simulink model "Extended_Model_1_1"  (R2024a)
settings: Solver=ode15s  StartTime=0.0  StopTime=100  FixedStep=0.0001  MaxStep=0.01  RelTol=1e-3  AbsTol=1e-3  EnableMultiTasking=on
model workspace (MATLAB code in the model file):
  | F_load_x= 2e3; %[N]
  | F_load_y= 1e4; %[N]
  | 
  | d=0.01;   %[m]
  | l=1;      %[m]
  | L=l;      %[m] Node distance
  | H=L*cos(pi/6); %[m] Node distance
  | 
  | Density=7800; %[kg/m^3]
  | E=210;   %[GPa]
  | G=79;    %[GPa]
  | bm=0.01; %[1/s]  Default
  | bk=0.01; %[s] Default
  | 
  | b_rj=1; %[N*m*s/rad] Damp.Coef.Revolut joints
  | 
  | Size_frame=30; %[pixel]
undefined symbols (not defined in the file): F_x, F_y, X, Y, Z
libraries: sm_lib x317, nesl_utility x64, fl_lib x6, simulink x1
(part 7 of 9)

== system Extended_Model_1_1/Subsystem4/Beam_4 ==
  note: Beam_D
  con : Inport
  Beam : sm_lib/Body Elements/Flexible Bodies/Beams/Flexible Cylindrical Beam  SectionType=Solid  Radius=d/2  RadiusUnits=m  Thickness=1  ThicknessUnits=mm  Length=l  LengthUnits=m  StiffnessAndInertiaType=CalculateFromGeometry  Density=Density  DensityUnits=kg/m^3  ModuliType=YoungsShear  YoungsModulus=E  YoungsModulusUnits=GPa  PoissonsRatio=0.28  ShearModulus=G  ShearModulusUnits=GPa  GeometricCentroid=[0 0]  GeometricCentroidUnits=m  BendingCentroid=[0 0]  BendingCentroidUnits=m  ShearCenter=[0 0]  ShearCenterUnits=m  AxialRigidity=1  AxialRigidityUnits=Pa*m^2  FlexuralRigidity=[1 1]  FlexuralRigidityUnits=Pa*m^4  CrossFlexuralRigidity=0  CrossFlexuralRigidityUnits=Pa*m^4  TorsionalRigidity=1  TorsionalRigidityUnits=Pa*m^4  CenterOfMass=[0 0]  CenterOfMassUnits=m  MassPerUnitLength=1  MassPerUnitLengthUnits=kg/m  MassMomentOfInertiaDensity=[1 1]  MassMomentOfInertiaDensityUnits=kg*m  MassProductOfInertiaDensity=0  MassProductOfInertiaDensityUnits=kg*m  DampingType=Proportional  ProportionalDampingAlpha=bm  ProportionalDampingAlphaUnits=1/s  ProportionalDampingBeta=bk  ProportionalDampingBetaUnits=s  UniformModalDampingRatio=0.01  NumElements=1  ReductionType=None  NumRetainedModes=1  GraphicType=FromGeometry  GraphicVisPropType=SimpleVisualProperties  GraphicDiffuseColor=[0.5 0.5 0.5]  GraphicOpacity=1.0  GraphicSpecularColor=[0.5 0.5 0.5 1.0]  GraphicAmbientColor=[0.15 0.15 0.15 1.0]  GraphicEmissiveColor=[0.0 0.0 0.0 1.0]  GraphicShininess=75  DoExposeZminFrame=on  DoExposeZmaxFrame=on  SerializedFrames=<Frames/>
      settings: AttributesFormatString=%<Description>
  Dot Product : DotProduct  OutDataTypeStr=Inherit: Inherit via internal rule
  Interpreted MATLAB Function : MATLABFcn  Description=u(3)  MATLABFcn=u(3)
      settings: AttributesFormatString=%<Description>
  PS-Simulink Converter6 : nesl_utility/PS-Simulink Converter  PhysicalDomain=network_engine_domain  SubClassName=ps_output  LeftPortType=input  RightPortType=output  PseudoPeriodic=off  Frequencies=[]  VectorFormat=inherit  Unit=1  AffineConversion=off
  Rigid Transform1 : sm_lib/Frames and Transforms/Rigid Transform  RotationMethod=StandardAxis  FollAlignAxisA=+X  BaseAlignAxisA=+Y  FollAlignAxisB=+Y  BaseAlignAxisB=+Z  RotationStandardAxis=+Y  RotationAngle=90  RotationAngleUnits=deg  RotationArbitraryAxis=[0 0 1]  RotationSequenceAxes=FollowerAxes  RotationSequence=XYX  RotationSequenceAngles=[0 0 0]  RotationSequenceAnglesUnits=deg  RotationMatrix=[1 0 0; 0 1 0; 0 0 1]  Quaternion=[1 0 0 0]  TranslationMethod=None  TranslationCartesianOffset=[0 0 0]  TranslationCartesianOffsetUnits=m  TranslationStandardAxis=+Z  TranslationStandardOffset=0  TranslationStandardOffsetUnits=m  TranslationROffset=0  TranslationROffsetUnits=m  TranslationThetaOffset=0  TranslationThetaOffsetUnits=deg  TranslationZOffset=0  TranslationZOffsetUnits=m
      settings: AttributesFormatString=|
      | %<RotationStandardAxis>
      | %<RotationAngle> deg
  Rigid Transform2 : sm_lib/Frames and Transforms/Rigid Transform  RotationMethod=StandardAxis  FollAlignAxisA=+X  BaseAlignAxisA=+Y  FollAlignAxisB=+Y  BaseAlignAxisB=+Z  RotationStandardAxis=+Y  RotationAngle=-90  RotationAngleUnits=deg  RotationArbitraryAxis=[0 0 1]  RotationSequenceAxes=FollowerAxes  RotationSequence=XYX  RotationSequenceAngles=[0 0 0]  RotationSequenceAnglesUnits=deg  RotationMatrix=[1 0 0; 0 1 0; 0 0 1]  Quaternion=[1 0 0 0]  TranslationMethod=None  TranslationCartesianOffset=[0 0 0]  TranslationCartesianOffsetUnits=m  TranslationStandardAxis=+Z  TranslationStandardOffset=0  TranslationStandardOffsetUnits=m  TranslationROffset=0  TranslationROffsetUnits=m  TranslationThetaOffset=0  TranslationThetaOffsetUnits=deg  TranslationZOffset=0  TranslationZOffsetUnits=m
      settings: AttributesFormatString=|
      | %<RotationStandardAxis>
      | %<RotationAngle> deg
  Weld Joint2 : sm_lib/Joints/Weld Joint  Description=|  JointMode=Normal  CompositeWrenchDir=FollowerOnBase  CompositeWrenchFrame=BaseFrame  SenseConstraintForce=off  SenseConstraintTorque=off  SenseTotalForce=on  SenseTotalTorque=off
      | Total force
      | sensing
      settings: AttributesFormatString=%<Description>
  B : PMIOPort  Side=Left
  F : PMIOPort  Port=2  Side=Right
  Ni : Outport
  wires:
  Interpreted MATLAB Function/1 -> Dot Product/1
  Dot Product/1 -> Ni/1
  con/1 -> Dot Product/2
  PS-Simulink Converter6/1 -> Interpreted MATLAB Function/1
  connections:
  Weld Joint2/RConn2 -- PS-Simulink Converter6/LConn1
  Rigid Transform1/LConn1 -- B/RConn1
  Beam/RConn1 -- Rigid Transform2/LConn1
  Rigid Transform2/RConn1 -- F/RConn1
  Weld Joint2/LConn1 -- Rigid Transform1/RConn1
  Beam/LConn1 -- Weld Joint2/RConn1

== system Extended_Model_1_1/Subsystem4/Subsystem ==
  Point Cloud1 : sm_lib/Curves and Surfaces/Point Cloud  Description=|  CoordinatesMatrix=[0 0 0]  CoordinatesMatrixUnits=m  GraphicType=MarkerCloud  GraphicSphereRadius=d/2  GraphicSphereRadiusUnits=m  GraphicVisPropType=SimpleVisualProperties  GraphicDiffuseColor=[0.5 0.5 0.5]  GraphicOpacity=1  GraphicSpecularColor=[0.5 0.5 0.5 1.0]  GraphicAmbientColor=[0.15 0.15 0.15 1.0]  GraphicEmissiveColor=[0.0 0.0 0.0 1.0]  GraphicShininess=75
      | Graphic
      | sphere
      settings: AttributesFormatString=%<Description>
  Point1 : sm_lib/Curves and Surfaces/Point  Description=|  GraphicType=Marker  MarkerShape=Frame  MarkerSize=Size_frame  GraphicVisPropType=SimpleVisualProperties  GraphicDiffuseColor=[0 1 0]  GraphicOpacity=1.0  GraphicSpecularColor=[0.5 0.5 0.5 1.0]  GraphicAmbientColor=[0.15 0.15 0.15 1.0]  GraphicEmissiveColor=[0.0 0.0 0.0 1.0]  GraphicShininess=75
      | Frame
      | visualization
      settings: AttributesFormatString=%<Description>
  Frame : PMIOPort  Side=Left
  connections:
  Point Cloud1/LConn1 -- Frame/RConn1 -- Point1/LConn1

== system Extended_Model_1_1/Subsystem4/Subsystem1 ==
  Point Cloud1 : sm_lib/Curves and Surfaces/Point Cloud  Description=|  CoordinatesMatrix=[0 0 0]  CoordinatesMatrixUnits=m  GraphicType=MarkerCloud  GraphicSphereRadius=d/2  GraphicSphereRadiusUnits=m  GraphicVisPropType=SimpleVisualProperties  GraphicDiffuseColor=[0.5 0.5 0.5]  GraphicOpacity=1  GraphicSpecularColor=[0.5 0.5 0.5 1.0]  GraphicAmbientColor=[0.15 0.15 0.15 1.0]  GraphicEmissiveColor=[0.0 0.0 0.0 1.0]  GraphicShininess=75
      | Graphic
      | sphere
      settings: AttributesFormatString=%<Description>
  Point1 : sm_lib/Curves and Surfaces/Point  Description=|  GraphicType=Marker  MarkerShape=Frame  MarkerSize=Size_frame  GraphicVisPropType=SimpleVisualProperties  GraphicDiffuseColor=[0 1 0]  GraphicOpacity=1.0  GraphicSpecularColor=[0.5 0.5 0.5 1.0]  GraphicAmbientColor=[0.15 0.15 0.15 1.0]  GraphicEmissiveColor=[0.0 0.0 0.0 1.0]  GraphicShininess=75
      | Frame
      | visualization
      settings: AttributesFormatString=%<Description>
  Frame : PMIOPort  Side=Left
  connections:
  Point Cloud1/LConn1 -- Frame/RConn1 -- Point1/LConn1

== system Extended_Model_1_1/Subsystem4/Subsystem2 ==
  Point Cloud1 : sm_lib/Curves and Surfaces/Point Cloud  Description=|  CoordinatesMatrix=[0 0 0]  CoordinatesMatrixUnits=m  GraphicType=MarkerCloud  GraphicSphereRadius=d/2  GraphicSphereRadiusUnits=m  GraphicVisPropType=SimpleVisualProperties  GraphicDiffuseColor=[0.5 0.5 0.5]  GraphicOpacity=1  GraphicSpecularColor=[0.5 0.5 0.5 1.0]  GraphicAmbientColor=[0.15 0.15 0.15 1.0]  GraphicEmissiveColor=[0.0 0.0 0.0 1.0]  GraphicShininess=75
      | Graphic
      | sphere
      settings: AttributesFormatString=%<Description>
  Point1 : sm_lib/Curves and Surfaces/Point  Description=|  GraphicType=Marker  MarkerShape=Frame  MarkerSize=Size_frame  GraphicVisPropType=SimpleVisualProperties  GraphicDiffuseColor=[0 1 0]  GraphicOpacity=1.0  GraphicSpecularColor=[0.5 0.5 0.5 1.0]  GraphicAmbientColor=[0.15 0.15 0.15 1.0]  GraphicEmissiveColor=[0.0 0.0 0.0 1.0]  GraphicShininess=75
      | Frame
      | visualization
      settings: AttributesFormatString=%<Description>
  Frame : PMIOPort  Side=Left
  connections:
  Point1/LConn1 -- Frame/RConn1 -- Point Cloud1/LConn1

== system Extended_Model_1_1/Subsystem5/Beam_1 ==
  note: Beam_A
  con : Inport
  Dot Product : DotProduct  OutDataTypeStr=Inherit: Inherit via internal rule
  Flexible Cylindrical Beam1 : sm_lib/Body Elements/Flexible Bodies/Beams/Flexible Cylindrical Beam  SectionType=Solid  Radius=d/2  RadiusUnits=m  Thickness=1  ThicknessUnits=mm  Length=l  LengthUnits=m  StiffnessAndInertiaType=CalculateFromGeometry  Density=Density  DensityUnits=kg/m^3  ModuliType=YoungsShear  YoungsModulus=E  YoungsModulusUnits=GPa  PoissonsRatio=0.28  ShearModulus=G  ShearModulusUnits=GPa  GeometricCentroid=[0 0]  GeometricCentroidUnits=m  BendingCentroid=[0 0]  BendingCentroidUnits=m  ShearCenter=[0 0]  ShearCenterUnits=m  AxialRigidity=1  AxialRigidityUnits=Pa*m^2  FlexuralRigidity=[1 1]  FlexuralRigidityUnits=Pa*m^4  CrossFlexuralRigidity=0  CrossFlexuralRigidityUnits=Pa*m^4  TorsionalRigidity=1  TorsionalRigidityUnits=Pa*m^4  CenterOfMass=[0 0]  CenterOfMassUnits=m  MassPerUnitLength=1  MassPerUnitLengthUnits=kg/m  MassMomentOfInertiaDensity=[1 1]  MassMomentOfInertiaDensityUnits=kg*m  MassProductOfInertiaDensity=0  MassProductOfInertiaDensityUnits=kg*m  DampingType=Proportional  ProportionalDampingAlpha=bm  ProportionalDampingAlphaUnits=1/s  ProportionalDampingBeta=bk  ProportionalDampingBetaUnits=s  UniformModalDampingRatio=0.01  NumElements=1  ReductionType=None  NumRetainedModes=1  GraphicType=FromGeometry  GraphicVisPropType=SimpleVisualProperties  GraphicDiffuseColor=[0.5 0.5 0.5]  GraphicOpacity=1.0  GraphicSpecularColor=[0.5 0.5 0.5 1.0]  GraphicAmbientColor=[0.15 0.15 0.15 1.0]  GraphicEmissiveColor=[0.0 0.0 0.0 1.0]  GraphicShininess=75  DoExposeZminFrame=on  DoExposeZmaxFrame=on  SerializedFrames=<Frames/>
      settings: AttributesFormatString=%<Description>
  Interpreted MATLAB Function : MATLABFcn  Description=u(3)  MATLABFcn=u(3)
      settings: AttributesFormatString=%<Description>
  PS-Simulink Converter6 : nesl_utility/PS-Simulink Converter  PhysicalDomain=network_engine_domain  SubClassName=ps_output  LeftPortType=input  RightPortType=output  PseudoPeriodic=off  Frequencies=[]  VectorFormat=inherit  Unit=1  AffineConversion=off
  Rigid Transform1 : sm_lib/Frames and Transforms/Rigid Transform  RotationMethod=StandardAxis  FollAlignAxisA=+X  BaseAlignAxisA=+Y  FollAlignAxisB=+Y  BaseAlignAxisB=+Z  RotationStandardAxis=+Y  RotationAngle=90  RotationAngleUnits=deg  RotationArbitraryAxis=[0 0 1]  RotationSequenceAxes=FollowerAxes  RotationSequence=XYX  RotationSequenceAngles=[0 0 0]  RotationSequenceAnglesUnits=deg  RotationMatrix=[1 0 0; 0 1 0; 0 0 1]  Quaternion=[1 0 0 0]  TranslationMethod=None  TranslationCartesianOffset=[0 0 0]  TranslationCartesianOffsetUnits=m  TranslationStandardAxis=+Z  TranslationStandardOffset=0  TranslationStandardOffsetUnits=m  TranslationROffset=0  TranslationROffsetUnits=m  TranslationThetaOffset=0  TranslationThetaOffsetUnits=deg  TranslationZOffset=0  TranslationZOffsetUnits=m
      settings: AttributesFormatString=|
      | %<RotationStandardAxis>
      | %<RotationAngle> deg
  Rigid Transform2 : sm_lib/Frames and Transforms/Rigid Transform  RotationMethod=StandardAxis  FollAlignAxisA=+X  BaseAlignAxisA=+Y  FollAlignAxisB=+Y  BaseAlignAxisB=+Z  RotationStandardAxis=+Y  RotationAngle=-90  RotationAngleUnits=deg  RotationArbitraryAxis=[0 0 1]  RotationSequenceAxes=FollowerAxes  RotationSequence=XYX  RotationSequenceAngles=[0 0 0]  RotationSequenceAnglesUnits=deg  RotationMatrix=[1 0 0; 0 1 0; 0 0 1]  Quaternion=[1 0 0 0]  TranslationMethod=None  TranslationCartesianOffset=[0 0 0]  TranslationCartesianOffsetUnits=m  TranslationStandardAxis=+Z  TranslationStandardOffset=0  TranslationStandardOffsetUnits=m  TranslationROffset=0  TranslationROffsetUnits=m  TranslationThetaOffset=0  TranslationThetaOffsetUnits=deg  TranslationZOffset=0  TranslationZOffsetUnits=m
      settings: AttributesFormatString=|
      | %<RotationStandardAxis>
      | %<RotationAngle> deg
  Weld Joint2 : sm_lib/Joints/Weld Joint  Description=|  JointMode=Normal  CompositeWrenchDir=FollowerOnBase  CompositeWrenchFrame=BaseFrame  SenseConstraintForce=off  SenseConstraintTorque=off  SenseTotalForce=on  SenseTotalTorque=off
      | Total force
      | sensing
      settings: AttributesFormatString=%<Description>
  B : PMIOPort  Side=Left
  F : PMIOPort  Port=2  Side=Right
  Ni : Outport
  wires:
  Interpreted MATLAB Function/1 -> Dot Product/1
  Dot Product/1 -> Ni/1
  PS-Simulink Converter6/1 -> Interpreted MATLAB Function/1
  con/1 -> Dot Product/2
  connections:
  Weld Joint2/LConn1 -- Rigid Transform1/RConn1
  Flexible Cylindrical Beam1/LConn1 -- Weld Joint2/RConn1
  Rigid Transform1/LConn1 -- B/RConn1
  Rigid Transform2/RConn1 -- F/RConn1
  Flexible Cylindrical Beam1/RConn1 -- Rigid Transform2/LConn1
  Weld Joint2/RConn2 -- PS-Simulink Converter6/LConn1

== system Extended_Model_1_1/Subsystem5/Beam_2 ==
  note: Beam_B
  con : Inport
  Dot Product : DotProduct  OutDataTypeStr=Inherit: Inherit via internal rule
  Flexible Cylindrical Beam1 : sm_lib/Body Elements/Flexible Bodies/Beams/Flexible Cylindrical Beam  SectionType=Solid  Radius=d/2  RadiusUnits=m  Thickness=1  ThicknessUnits=mm  Length=l  LengthUnits=m  StiffnessAndInertiaType=CalculateFromGeometry  Density=Density  DensityUnits=kg/m^3  ModuliType=YoungsShear  YoungsModulus=E  YoungsModulusUnits=GPa  PoissonsRatio=0.28  ShearModulus=G  ShearModulusUnits=GPa  GeometricCentroid=[0 0]  GeometricCentroidUnits=m  BendingCentroid=[0 0]  BendingCentroidUnits=m  ShearCenter=[0 0]  ShearCenterUnits=m  AxialRigidity=1  AxialRigidityUnits=Pa*m^2  FlexuralRigidity=[1 1]  FlexuralRigidityUnits=Pa*m^4  CrossFlexuralRigidity=0  CrossFlexuralRigidityUnits=Pa*m^4  TorsionalRigidity=1  TorsionalRigidityUnits=Pa*m^4  CenterOfMass=[0 0]  CenterOfMassUnits=m  MassPerUnitLength=1  MassPerUnitLengthUnits=kg/m  MassMomentOfInertiaDensity=[1 1]  MassMomentOfInertiaDensityUnits=kg*m  MassProductOfInertiaDensity=0  MassProductOfInertiaDensityUnits=kg*m  DampingType=Proportional  ProportionalDampingAlpha=bm  ProportionalDampingAlphaUnits=1/s  ProportionalDampingBeta=bk  ProportionalDampingBetaUnits=s  UniformModalDampingRatio=0.01  NumElements=1  ReductionType=None  NumRetainedModes=1  GraphicType=FromGeometry  GraphicVisPropType=SimpleVisualProperties  GraphicDiffuseColor=[0.5 0.5 0.5]  GraphicOpacity=1.0  GraphicSpecularColor=[0.5 0.5 0.5 1.0]  GraphicAmbientColor=[0.15 0.15 0.15 1.0]  GraphicEmissiveColor=[0.0 0.0 0.0 1.0]  GraphicShininess=75  DoExposeZminFrame=on  DoExposeZmaxFrame=on  SerializedFrames=<Frames/>
      settings: AttributesFormatString=%<Description>
  Interpreted MATLAB Function : MATLABFcn  Description=u(3)  MATLABFcn=u(3)
      settings: AttributesFormatString=%<Description>
  PS-Simulink Converter6 : nesl_utility/PS-Simulink Converter  PhysicalDomain=network_engine_domain  SubClassName=ps_output  LeftPortType=input  RightPortType=output  PseudoPeriodic=off  Frequencies=[]  VectorFormat=inherit  Unit=1  AffineConversion=off
  Rigid Transform1 : sm_lib/Frames and Transforms/Rigid Transform  RotationMethod=StandardAxis  FollAlignAxisA=+X  BaseAlignAxisA=+Y  FollAlignAxisB=+Y  BaseAlignAxisB=+Z  RotationStandardAxis=+Y  RotationAngle=90  RotationAngleUnits=deg  RotationArbitraryAxis=[0 0 1]  RotationSequenceAxes=FollowerAxes  RotationSequence=XYX  RotationSequenceAngles=[0 0 0]  RotationSequenceAnglesUnits=deg  RotationMatrix=[1 0 0; 0 1 0; 0 0 1]  Quaternion=[1 0 0 0]  TranslationMethod=None  TranslationCartesianOffset=[0 0 0]  TranslationCartesianOffsetUnits=m  TranslationStandardAxis=+Z  TranslationStandardOffset=0  TranslationStandardOffsetUnits=m  TranslationROffset=0  TranslationROffsetUnits=m  TranslationThetaOffset=0  TranslationThetaOffsetUnits=deg  TranslationZOffset=0  TranslationZOffsetUnits=m
      settings: AttributesFormatString=|
      | %<RotationStandardAxis>
      | %<RotationAngle> deg
  Rigid Transform2 : sm_lib/Frames and Transforms/Rigid Transform  RotationMethod=StandardAxis  FollAlignAxisA=+X  BaseAlignAxisA=+Y  FollAlignAxisB=+Y  BaseAlignAxisB=+Z  RotationStandardAxis=+Y  RotationAngle=-90  RotationAngleUnits=deg  RotationArbitraryAxis=[0 0 1]  RotationSequenceAxes=FollowerAxes  RotationSequence=XYX  RotationSequenceAngles=[0 0 0]  RotationSequenceAnglesUnits=deg  RotationMatrix=[1 0 0; 0 1 0; 0 0 1]  Quaternion=[1 0 0 0]  TranslationMethod=None  TranslationCartesianOffset=[0 0 0]  TranslationCartesianOffsetUnits=m  TranslationStandardAxis=+Z  TranslationStandardOffset=0  TranslationStandardOffsetUnits=m  TranslationROffset=0  TranslationROffsetUnits=m  TranslationThetaOffset=0  TranslationThetaOffsetUnits=deg  TranslationZOffset=0  TranslationZOffsetUnits=m
      settings: AttributesFormatString=|
      | %<RotationStandardAxis>
      | %<RotationAngle> deg
  Weld Joint2 : sm_lib/Joints/Weld Joint  Description=|  JointMode=Normal  CompositeWrenchDir=FollowerOnBase  CompositeWrenchFrame=BaseFrame  SenseConstraintForce=off  SenseConstraintTorque=off  SenseTotalForce=on  SenseTotalTorque=off
      | Total force
      | sensing
      settings: AttributesFormatString=%<Description>
  B : PMIOPort  Side=Left
  F : PMIOPort  Port=2  Side=Right
  Ni : Outport
  wires:
  con/1 -> Dot Product/2
  PS-Simulink Converter6/1 -> Interpreted MATLAB Function/1
  Dot Product/1 -> Ni/1
  Interpreted MATLAB Function/1 -> Dot Product/1
  connections:
  Weld Joint2/RConn2 -- PS-Simulink Converter6/LConn1
  Flexible Cylindrical Beam1/RConn1 -- Rigid Transform2/LConn1
  Rigid Transform2/RConn1 -- F/RConn1
  Rigid Transform1/LConn1 -- B/RConn1
  Flexible Cylindrical Beam1/LConn1 -- Weld Joint2/RConn1
  Weld Joint2/LConn1 -- Rigid Transform1/RConn1

== system Extended_Model_1_1/Subsystem5/Beam_3 ==
  note: Beam_C
  con : Inport
  Beam : sm_lib/Body Elements/Flexible Bodies/Beams/Flexible Cylindrical Beam  SectionType=Solid  Radius=d/2  RadiusUnits=m  Thickness=1  ThicknessUnits=mm  Length=l  LengthUnits=m  StiffnessAndInertiaType=CalculateFromGeometry  Density=Density  DensityUnits=kg/m^3  ModuliType=YoungsShear  YoungsModulus=E  YoungsModulusUnits=GPa  PoissonsRatio=0.28  ShearModulus=G  ShearModulusUnits=GPa  GeometricCentroid=[0 0]  GeometricCentroidUnits=m  BendingCentroid=[0 0]  BendingCentroidUnits=m  ShearCenter=[0 0]  ShearCenterUnits=m  AxialRigidity=1  AxialRigidityUnits=Pa*m^2  FlexuralRigidity=[1 1]  FlexuralRigidityUnits=Pa*m^4  CrossFlexuralRigidity=0  CrossFlexuralRigidityUnits=Pa*m^4  TorsionalRigidity=1  TorsionalRigidityUnits=Pa*m^4  CenterOfMass=[0 0]  CenterOfMassUnits=m  MassPerUnitLength=1  MassPerUnitLengthUnits=kg/m  MassMomentOfInertiaDensity=[1 1]  MassMomentOfInertiaDensityUnits=kg*m  MassProductOfInertiaDensity=0  MassProductOfInertiaDensityUnits=kg*m  DampingType=Proportional  ProportionalDampingAlpha=bm  ProportionalDampingAlphaUnits=1/s  ProportionalDampingBeta=bk  ProportionalDampingBetaUnits=s  UniformModalDampingRatio=0.01  NumElements=1  ReductionType=None  NumRetainedModes=1  GraphicType=FromGeometry  GraphicVisPropType=SimpleVisualProperties  GraphicDiffuseColor=[0.5 0.5 0.5]  GraphicOpacity=1.0  GraphicSpecularColor=[0.5 0.5 0.5 1.0]  GraphicAmbientColor=[0.15 0.15 0.15 1.0]  GraphicEmissiveColor=[0.0 0.0 0.0 1.0]  GraphicShininess=75  DoExposeZminFrame=on  DoExposeZmaxFrame=on  SerializedFrames=<Frames/>
      settings: AttributesFormatString=%<Description>
  Dot Product : DotProduct  OutDataTypeStr=Inherit: Inherit via internal rule
  Interpreted MATLAB Function : MATLABFcn  Description=u(3)  MATLABFcn=u(3)
      settings: AttributesFormatString=%<Description>
  PS-Simulink Converter6 : nesl_utility/PS-Simulink Converter  PhysicalDomain=network_engine_domain  SubClassName=ps_output  LeftPortType=input  RightPortType=output  PseudoPeriodic=off  Frequencies=[]  VectorFormat=inherit  Unit=1  AffineConversion=off
  Rigid Transform1 : sm_lib/Frames and Transforms/Rigid Transform  RotationMethod=StandardAxis  FollAlignAxisA=+X  BaseAlignAxisA=+Y  FollAlignAxisB=+Y  BaseAlignAxisB=+Z  RotationStandardAxis=+Y  RotationAngle=90  RotationAngleUnits=deg  RotationArbitraryAxis=[0 0 1]  RotationSequenceAxes=FollowerAxes  RotationSequence=XYX  RotationSequenceAngles=[0 0 0]  RotationSequenceAnglesUnits=deg  RotationMatrix=[1 0 0; 0 1 0; 0 0 1]  Quaternion=[1 0 0 0]  TranslationMethod=None  TranslationCartesianOffset=[0 0 0]  TranslationCartesianOffsetUnits=m  TranslationStandardAxis=+Z  TranslationStandardOffset=0  TranslationStandardOffsetUnits=m  TranslationROffset=0  TranslationROffsetUnits=m  TranslationThetaOffset=0  TranslationThetaOffsetUnits=deg  TranslationZOffset=0  TranslationZOffsetUnits=m
      settings: AttributesFormatString=|
      | %<RotationStandardAxis>
      | %<RotationAngle> deg
  Rigid Transform2 : sm_lib/Frames and Transforms/Rigid Transform  RotationMethod=StandardAxis  FollAlignAxisA=+X  BaseAlignAxisA=+Y  FollAlignAxisB=+Y  BaseAlignAxisB=+Z  RotationStandardAxis=+Y  RotationAngle=-90  RotationAngleUnits=deg  RotationArbitraryAxis=[0 0 1]  RotationSequenceAxes=FollowerAxes  RotationSequence=XYX  RotationSequenceAngles=[0 0 0]  RotationSequenceAnglesUnits=deg  RotationMatrix=[1 0 0; 0 1 0; 0 0 1]  Quaternion=[1 0 0 0]  TranslationMethod=None  TranslationCartesianOffset=[0 0 0]  TranslationCartesianOffsetUnits=m  TranslationStandardAxis=+Z  TranslationStandardOffset=0  TranslationStandardOffsetUnits=m  TranslationROffset=0  TranslationROffsetUnits=m  TranslationThetaOffset=0  TranslationThetaOffsetUnits=deg  TranslationZOffset=0  TranslationZOffsetUnits=m
      settings: AttributesFormatString=|
      | %<RotationStandardAxis>
      | %<RotationAngle> deg
  Weld Joint2 : sm_lib/Joints/Weld Joint  Description=|  JointMode=Normal  CompositeWrenchDir=FollowerOnBase  CompositeWrenchFrame=BaseFrame  SenseConstraintForce=off  SenseConstraintTorque=off  SenseTotalForce=on  SenseTotalTorque=off
      | Total force
      | sensing
      settings: AttributesFormatString=%<Description>
  B : PMIOPort  Side=Left
  F : PMIOPort  Port=2  Side=Right
  Ni : Outport
  wires:
  PS-Simulink Converter6/1 -> Interpreted MATLAB Function/1
  con/1 -> Dot Product/2
  Dot Product/1 -> Ni/1
  Interpreted MATLAB Function/1 -> Dot Product/1
  connections:
  Beam/LConn1 -- Weld Joint2/RConn1
  Weld Joint2/LConn1 -- Rigid Transform1/RConn1
  Rigid Transform2/RConn1 -- F/RConn1
  Beam/RConn1 -- Rigid Transform2/LConn1
  Rigid Transform1/LConn1 -- B/RConn1
  Weld Joint2/RConn2 -- PS-Simulink Converter6/LConn1

== system Extended_Model_1_1/Subsystem5/Beam_4 ==
  note: Beam_D
  con : Inport
  Beam : sm_lib/Body Elements/Flexible Bodies/Beams/Flexible Cylindrical Beam  SectionType=Solid  Radius=d/2  RadiusUnits=m  Thickness=1  ThicknessUnits=mm  Length=l  LengthUnits=m  StiffnessAndInertiaType=CalculateFromGeometry  Density=Density  DensityUnits=kg/m^3  ModuliType=YoungsShear  YoungsModulus=E  YoungsModulusUnits=GPa  PoissonsRatio=0.28  ShearModulus=G  ShearModulusUnits=GPa  GeometricCentroid=[0 0]  GeometricCentroidUnits=m  BendingCentroid=[0 0]  BendingCentroidUnits=m  ShearCenter=[0 0]  ShearCenterUnits=m  AxialRigidity=1  AxialRigidityUnits=Pa*m^2  FlexuralRigidity=[1 1]  FlexuralRigidityUnits=Pa*m^4  CrossFlexuralRigidity=0  CrossFlexuralRigidityUnits=Pa*m^4  TorsionalRigidity=1  TorsionalRigidityUnits=Pa*m^4  CenterOfMass=[0 0]  CenterOfMassUnits=m  MassPerUnitLength=1  MassPerUnitLengthUnits=kg/m  MassMomentOfInertiaDensity=[1 1]  MassMomentOfInertiaDensityUnits=kg*m  MassProductOfInertiaDensity=0  MassProductOfInertiaDensityUnits=kg*m  DampingType=Proportional  ProportionalDampingAlpha=bm  ProportionalDampingAlphaUnits=1/s  ProportionalDampingBeta=bk  ProportionalDampingBetaUnits=s  UniformModalDampingRatio=0.01  NumElements=1  ReductionType=None  NumRetainedModes=1  GraphicType=FromGeometry  GraphicVisPropType=SimpleVisualProperties  GraphicDiffuseColor=[0.5 0.5 0.5]  GraphicOpacity=1.0  GraphicSpecularColor=[0.5 0.5 0.5 1.0]  GraphicAmbientColor=[0.15 0.15 0.15 1.0]  GraphicEmissiveColor=[0.0 0.0 0.0 1.0]  GraphicShininess=75  DoExposeZminFrame=on  DoExposeZmaxFrame=on  SerializedFrames=<Frames/>
      settings: AttributesFormatString=%<Description>
  Dot Product : DotProduct  OutDataTypeStr=Inherit: Inherit via internal rule
  Interpreted MATLAB Function : MATLABFcn  Description=u(3)  MATLABFcn=u(3)
      settings: AttributesFormatString=%<Description>
  PS-Simulink Converter6 : nesl_utility/PS-Simulink Converter  PhysicalDomain=network_engine_domain  SubClassName=ps_output  LeftPortType=input  RightPortType=output  PseudoPeriodic=off  Frequencies=[]  VectorFormat=inherit  Unit=1  AffineConversion=off
  Rigid Transform1 : sm_lib/Frames and Transforms/Rigid Transform  RotationMethod=StandardAxis  FollAlignAxisA=+X  BaseAlignAxisA=+Y  FollAlignAxisB=+Y  BaseAlignAxisB=+Z  RotationStandardAxis=+Y  RotationAngle=90  RotationAngleUnits=deg  RotationArbitraryAxis=[0 0 1]  RotationSequenceAxes=FollowerAxes  RotationSequence=XYX  RotationSequenceAngles=[0 0 0]  RotationSequenceAnglesUnits=deg  RotationMatrix=[1 0 0; 0 1 0; 0 0 1]  Quaternion=[1 0 0 0]  TranslationMethod=None  TranslationCartesianOffset=[0 0 0]  TranslationCartesianOffsetUnits=m  TranslationStandardAxis=+Z  TranslationStandardOffset=0  TranslationStandardOffsetUnits=m  TranslationROffset=0  TranslationROffsetUnits=m  TranslationThetaOffset=0  TranslationThetaOffsetUnits=deg  TranslationZOffset=0  TranslationZOffsetUnits=m
      settings: AttributesFormatString=|
      | %<RotationStandardAxis>
      | %<RotationAngle> deg
  Rigid Transform2 : sm_lib/Frames and Transforms/Rigid Transform  RotationMethod=StandardAxis  FollAlignAxisA=+X  BaseAlignAxisA=+Y  FollAlignAxisB=+Y  BaseAlignAxisB=+Z  RotationStandardAxis=+Y  RotationAngle=-90  RotationAngleUnits=deg  RotationArbitraryAxis=[0 0 1]  RotationSequenceAxes=FollowerAxes  RotationSequence=XYX  RotationSequenceAngles=[0 0 0]  RotationSequenceAnglesUnits=deg  RotationMatrix=[1 0 0; 0 1 0; 0 0 1]  Quaternion=[1 0 0 0]  TranslationMethod=None  TranslationCartesianOffset=[0 0 0]  TranslationCartesianOffsetUnits=m  TranslationStandardAxis=+Z  TranslationStandardOffset=0  TranslationStandardOffsetUnits=m  TranslationROffset=0  TranslationROffsetUnits=m  TranslationThetaOffset=0  TranslationThetaOffsetUnits=deg  TranslationZOffset=0  TranslationZOffsetUnits=m
      settings: AttributesFormatString=|
      | %<RotationStandardAxis>
      | %<RotationAngle> deg
  Weld Joint2 : sm_lib/Joints/Weld Joint  Description=|  JointMode=Normal  CompositeWrenchDir=FollowerOnBase  CompositeWrenchFrame=BaseFrame  SenseConstraintForce=off  SenseConstraintTorque=off  SenseTotalForce=on  SenseTotalTorque=off
      | Total force
      | sensing
      settings: AttributesFormatString=%<Description>
  B : PMIOPort  Side=Left
  F : PMIOPort  Port=2  Side=Right
  Ni : Outport
  wires:
  PS-Simulink Converter6/1 -> Interpreted MATLAB Function/1
  con/1 -> Dot Product/2
  Dot Product/1 -> Ni/1
  Interpreted MATLAB Function/1 -> Dot Product/1
  connections:
  Beam/LConn1 -- Weld Joint2/RConn1
  Weld Joint2/LConn1 -- Rigid Transform1/RConn1
  Rigid Transform2/RConn1 -- F/RConn1
  Beam/RConn1 -- Rigid Transform2/LConn1
  Rigid Transform1/LConn1 -- B/RConn1
  Weld Joint2/RConn2 -- PS-Simulink Converter6/LConn1

== system Extended_Model_1_1/Subsystem5/Subsystem ==
  Point Cloud1 : sm_lib/Curves and Surfaces/Point Cloud  Description=|  CoordinatesMatrix=[0 0 0]  CoordinatesMatrixUnits=m  GraphicType=MarkerCloud  GraphicSphereRadius=d/2  GraphicSphereRadiusUnits=m  GraphicVisPropType=SimpleVisualProperties  GraphicDiffuseColor=[0.5 0.5 0.5]  GraphicOpacity=1  GraphicSpecularColor=[0.5 0.5 0.5 1.0]  GraphicAmbientColor=[0.15 0.15 0.15 1.0]  GraphicEmissiveColor=[0.0 0.0 0.0 1.0]  GraphicShininess=75
      | Graphic
      | sphere
      settings: AttributesFormatString=%<Description>
  Point1 : sm_lib/Curves and Surfaces/Point  Description=|  GraphicType=Marker  MarkerShape=Frame  MarkerSize=Size_frame  GraphicVisPropType=SimpleVisualProperties  GraphicDiffuseColor=[0 1 0]  GraphicOpacity=1.0  GraphicSpecularColor=[0.5 0.5 0.5 1.0]  GraphicAmbientColor=[0.15 0.15 0.15 1.0]  GraphicEmissiveColor=[0.0 0.0 0.0 1.0]  GraphicShininess=75
      | Frame
      | visualization
      settings: AttributesFormatString=%<Description>
  Frame : PMIOPort  Side=Left
  connections:
  Point1/LConn1 -- Frame/RConn1 -- Point Cloud1/LConn1

== system Extended_Model_1_1/Subsystem5/Subsystem1 ==
  Point Cloud1 : sm_lib/Curves and Surfaces/Point Cloud  Description=|  CoordinatesMatrix=[0 0 0]  CoordinatesMatrixUnits=m  GraphicType=MarkerCloud  GraphicSphereRadius=d/2  GraphicSphereRadiusUnits=m  GraphicVisPropType=SimpleVisualProperties  GraphicDiffuseColor=[0.5 0.5 0.5]  GraphicOpacity=1  GraphicSpecularColor=[0.5 0.5 0.5 1.0]  GraphicAmbientColor=[0.15 0.15 0.15 1.0]  GraphicEmissiveColor=[0.0 0.0 0.0 1.0]  GraphicShininess=75
      | Graphic
      | sphere
      settings: AttributesFormatString=%<Description>
  Point1 : sm_lib/Curves and Surfaces/Point  Description=|  GraphicType=Marker  MarkerShape=Frame  MarkerSize=Size_frame  GraphicVisPropType=SimpleVisualProperties  GraphicDiffuseColor=[0 1 0]  GraphicOpacity=1.0  GraphicSpecularColor=[0.5 0.5 0.5 1.0]  GraphicAmbientColor=[0.15 0.15 0.15 1.0]  GraphicEmissiveColor=[0.0 0.0 0.0 1.0]  GraphicShininess=75
      | Frame
      | visualization
      settings: AttributesFormatString=%<Description>
  Frame : PMIOPort  Side=Left
  connections:
  Point1/LConn1 -- Frame/RConn1 -- Point Cloud1/LConn1

== system Extended_Model_1_1/Subsystem5/Subsystem2 ==
  Point Cloud1 : sm_lib/Curves and Surfaces/Point Cloud  Description=|  CoordinatesMatrix=[0 0 0]  CoordinatesMatrixUnits=m  GraphicType=MarkerCloud  GraphicSphereRadius=d/2  GraphicSphereRadiusUnits=m  GraphicVisPropType=SimpleVisualProperties  GraphicDiffuseColor=[0.5 0.5 0.5]  GraphicOpacity=1  GraphicSpecularColor=[0.5 0.5 0.5 1.0]  GraphicAmbientColor=[0.15 0.15 0.15 1.0]  GraphicEmissiveColor=[0.0 0.0 0.0 1.0]  GraphicShininess=75
      | Graphic
      | sphere
      settings: AttributesFormatString=%<Description>
  Point1 : sm_lib/Curves and Surfaces/Point  Description=|  GraphicType=Marker  MarkerShape=Frame  MarkerSize=Size_frame  GraphicVisPropType=SimpleVisualProperties  GraphicDiffuseColor=[0 1 0]  GraphicOpacity=1.0  GraphicSpecularColor=[0.5 0.5 0.5 1.0]  GraphicAmbientColor=[0.15 0.15 0.15 1.0]  GraphicEmissiveColor=[0.0 0.0 0.0 1.0]  GraphicShininess=75
      | Frame
      | visualization
      settings: AttributesFormatString=%<Description>
  Frame : PMIOPort  Side=Left
  connections:
  Point Cloud1/LConn1 -- Frame/RConn1 -- Point1/LConn1

== system Extended_Model_1_1/Subsystem6/Beam_1 ==
  note: Beam_A
  con : Inport
  Dot Product : DotProduct  OutDataTypeStr=Inherit: Inherit via internal rule
  Flexible Cylindrical Beam1 : sm_lib/Body Elements/Flexible Bodies/Beams/Flexible Cylindrical Beam  SectionType=Solid  Radius=d/2  RadiusUnits=m  Thickness=1  ThicknessUnits=mm  Length=l  LengthUnits=m  StiffnessAndInertiaType=CalculateFromGeometry  Density=Density  DensityUnits=kg/m^3  ModuliType=YoungsShear  YoungsModulus=E  YoungsModulusUnits=GPa  PoissonsRatio=0.28  ShearModulus=G  ShearModulusUnits=GPa  GeometricCentroid=[0 0]  GeometricCentroidUnits=m  BendingCentroid=[0 0]  BendingCentroidUnits=m  ShearCenter=[0 0]  ShearCenterUnits=m  AxialRigidity=1  AxialRigidityUnits=Pa*m^2  FlexuralRigidity=[1 1]  FlexuralRigidityUnits=Pa*m^4  CrossFlexuralRigidity=0  CrossFlexuralRigidityUnits=Pa*m^4  TorsionalRigidity=1  TorsionalRigidityUnits=Pa*m^4  CenterOfMass=[0 0]  CenterOfMassUnits=m  MassPerUnitLength=1  MassPerUnitLengthUnits=kg/m  MassMomentOfInertiaDensity=[1 1]  MassMomentOfInertiaDensityUnits=kg*m  MassProductOfInertiaDensity=0  MassProductOfInertiaDensityUnits=kg*m  DampingType=Proportional  ProportionalDampingAlpha=bm  ProportionalDampingAlphaUnits=1/s  ProportionalDampingBeta=bk  ProportionalDampingBetaUnits=s  UniformModalDampingRatio=0.01  NumElements=1  ReductionType=None  NumRetainedModes=1  GraphicType=FromGeometry  GraphicVisPropType=SimpleVisualProperties  GraphicDiffuseColor=[0.5 0.5 0.5]  GraphicOpacity=1.0  GraphicSpecularColor=[0.5 0.5 0.5 1.0]  GraphicAmbientColor=[0.15 0.15 0.15 1.0]  GraphicEmissiveColor=[0.0 0.0 0.0 1.0]  GraphicShininess=75  DoExposeZminFrame=on  DoExposeZmaxFrame=on  SerializedFrames=<Frames/>
      settings: AttributesFormatString=%<Description>
  Interpreted MATLAB Function : MATLABFcn  Description=u(3)  MATLABFcn=u(3)
      settings: AttributesFormatString=%<Description>
  PS-Simulink Converter6 : nesl_utility/PS-Simulink Converter  PhysicalDomain=network_engine_domain  SubClassName=ps_output  LeftPortType=input  RightPortType=output  PseudoPeriodic=off  Frequencies=[]  VectorFormat=inherit  Unit=1  AffineConversion=off
  Rigid Transform1 : sm_lib/Frames and Transforms/Rigid Transform  RotationMethod=StandardAxis  FollAlignAxisA=+X  BaseAlignAxisA=+Y  FollAlignAxisB=+Y  BaseAlignAxisB=+Z  RotationStandardAxis=+Y  RotationAngle=90  RotationAngleUnits=deg  RotationArbitraryAxis=[0 0 1]  RotationSequenceAxes=FollowerAxes  RotationSequence=XYX  RotationSequenceAngles=[0 0 0]  RotationSequenceAnglesUnits=deg  RotationMatrix=[1 0 0; 0 1 0; 0 0 1]  Quaternion=[1 0 0 0]  TranslationMethod=None  TranslationCartesianOffset=[0 0 0]  TranslationCartesianOffsetUnits=m  TranslationStandardAxis=+Z  TranslationStandardOffset=0  TranslationStandardOffsetUnits=m  TranslationROffset=0  TranslationROffsetUnits=m  TranslationThetaOffset=0  TranslationThetaOffsetUnits=deg  TranslationZOffset=0  TranslationZOffsetUnits=m
      settings: AttributesFormatString=|
      | %<RotationStandardAxis>
      | %<RotationAngle> deg
  Rigid Transform2 : sm_lib/Frames and Transforms/Rigid Transform  RotationMethod=StandardAxis  FollAlignAxisA=+X  BaseAlignAxisA=+Y  FollAlignAxisB=+Y  BaseAlignAxisB=+Z  RotationStandardAxis=+Y  RotationAngle=-90  RotationAngleUnits=deg  RotationArbitraryAxis=[0 0 1]  RotationSequenceAxes=FollowerAxes  RotationSequence=XYX  RotationSequenceAngles=[0 0 0]  RotationSequenceAnglesUnits=deg  RotationMatrix=[1 0 0; 0 1 0; 0 0 1]  Quaternion=[1 0 0 0]  TranslationMethod=None  TranslationCartesianOffset=[0 0 0]  TranslationCartesianOffsetUnits=m  TranslationStandardAxis=+Z  TranslationStandardOffset=0  TranslationStandardOffsetUnits=m  TranslationROffset=0  TranslationROffsetUnits=m  TranslationThetaOffset=0  TranslationThetaOffsetUnits=deg  TranslationZOffset=0  TranslationZOffsetUnits=m
      settings: AttributesFormatString=|
      | %<RotationStandardAxis>
      | %<RotationAngle> deg
  Weld Joint2 : sm_lib/Joints/Weld Joint  Description=|  JointMode=Normal  CompositeWrenchDir=FollowerOnBase  CompositeWrenchFrame=BaseFrame  SenseConstraintForce=off  SenseConstraintTorque=off  SenseTotalForce=on  SenseTotalTorque=off
      | Total force
      | sensing
      settings: AttributesFormatString=%<Description>
  B : PMIOPort  Side=Left
  F : PMIOPort  Port=2  Side=Right
  Ni : Outport
  wires:
  con/1 -> Dot Product/2
  PS-Simulink Converter6/1 -> Interpreted MATLAB Function/1
  Dot Product/1 -> Ni/1
  Interpreted MATLAB Function/1 -> Dot Product/1
  connections:
  Weld Joint2/RConn2 -- PS-Simulink Converter6/LConn1
  Flexible Cylindrical Beam1/RConn1 -- Rigid Transform2/LConn1
  Rigid Transform2/RConn1 -- F/RConn1
  Rigid Transform1/LConn1 -- B/RConn1
  Flexible Cylindrical Beam1/LConn1 -- Weld Joint2/RConn1
  Weld Joint2/LConn1 -- Rigid Transform1/RConn1

== system Extended_Model_1_1/Subsystem6/Beam_2 ==
  note: Beam_B
  con : Inport
  Dot Product : DotProduct  OutDataTypeStr=Inherit: Inherit via internal rule
  Flexible Cylindrical Beam1 : sm_lib/Body Elements/Flexible Bodies/Beams/Flexible Cylindrical Beam  SectionType=Solid  Radius=d/2  RadiusUnits=m  Thickness=1  ThicknessUnits=mm  Length=l  LengthUnits=m  StiffnessAndInertiaType=CalculateFromGeometry  Density=Density  DensityUnits=kg/m^3  ModuliType=YoungsShear  YoungsModulus=E  YoungsModulusUnits=GPa  PoissonsRatio=0.28  ShearModulus=G  ShearModulusUnits=GPa  GeometricCentroid=[0 0]  GeometricCentroidUnits=m  BendingCentroid=[0 0]  BendingCentroidUnits=m  ShearCenter=[0 0]  ShearCenterUnits=m  AxialRigidity=1  AxialRigidityUnits=Pa*m^2  FlexuralRigidity=[1 1]  FlexuralRigidityUnits=Pa*m^4  CrossFlexuralRigidity=0  CrossFlexuralRigidityUnits=Pa*m^4  TorsionalRigidity=1  TorsionalRigidityUnits=Pa*m^4  CenterOfMass=[0 0]  CenterOfMassUnits=m  MassPerUnitLength=1  MassPerUnitLengthUnits=kg/m  MassMomentOfInertiaDensity=[1 1]  MassMomentOfInertiaDensityUnits=kg*m  MassProductOfInertiaDensity=0  MassProductOfInertiaDensityUnits=kg*m  DampingType=Proportional  ProportionalDampingAlpha=bm  ProportionalDampingAlphaUnits=1/s  ProportionalDampingBeta=bk  ProportionalDampingBetaUnits=s  UniformModalDampingRatio=0.01  NumElements=1  ReductionType=None  NumRetainedModes=1  GraphicType=FromGeometry  GraphicVisPropType=SimpleVisualProperties  GraphicDiffuseColor=[0.5 0.5 0.5]  GraphicOpacity=1.0  GraphicSpecularColor=[0.5 0.5 0.5 1.0]  GraphicAmbientColor=[0.15 0.15 0.15 1.0]  GraphicEmissiveColor=[0.0 0.0 0.0 1.0]  GraphicShininess=75  DoExposeZminFrame=on  DoExposeZmaxFrame=on  SerializedFrames=<Frames/>
      settings: AttributesFormatString=%<Description>
  Interpreted MATLAB Function : MATLABFcn  Description=u(3)  MATLABFcn=u(3)
      settings: AttributesFormatString=%<Description>
  PS-Simulink Converter6 : nesl_utility/PS-Simulink Converter  PhysicalDomain=network_engine_domain  SubClassName=ps_output  LeftPortType=input  RightPortType=output  PseudoPeriodic=off  Frequencies=[]  VectorFormat=inherit  Unit=1  AffineConversion=off
  Rigid Transform1 : sm_lib/Frames and Transforms/Rigid Transform  RotationMethod=StandardAxis  FollAlignAxisA=+X  BaseAlignAxisA=+Y  FollAlignAxisB=+Y  BaseAlignAxisB=+Z  RotationStandardAxis=+Y  RotationAngle=90  RotationAngleUnits=deg  RotationArbitraryAxis=[0 0 1]  RotationSequenceAxes=FollowerAxes  RotationSequence=XYX  RotationSequenceAngles=[0 0 0]  RotationSequenceAnglesUnits=deg  RotationMatrix=[1 0 0; 0 1 0; 0 0 1]  Quaternion=[1 0 0 0]  TranslationMethod=None  TranslationCartesianOffset=[0 0 0]  TranslationCartesianOffsetUnits=m  TranslationStandardAxis=+Z  TranslationStandardOffset=0  TranslationStandardOffsetUnits=m  TranslationROffset=0  TranslationROffsetUnits=m  TranslationThetaOffset=0  TranslationThetaOffsetUnits=deg  TranslationZOffset=0  TranslationZOffsetUnits=m
      settings: AttributesFormatString=|
      | %<RotationStandardAxis>
      | %<RotationAngle> deg
  Rigid Transform2 : sm_lib/Frames and Transforms/Rigid Transform  RotationMethod=StandardAxis  FollAlignAxisA=+X  BaseAlignAxisA=+Y  FollAlignAxisB=+Y  BaseAlignAxisB=+Z  RotationStandardAxis=+Y  RotationAngle=-90  RotationAngleUnits=deg  RotationArbitraryAxis=[0 0 1]  RotationSequenceAxes=FollowerAxes  RotationSequence=XYX  RotationSequenceAngles=[0 0 0]  RotationSequenceAnglesUnits=deg  RotationMatrix=[1 0 0; 0 1 0; 0 0 1]  Quaternion=[1 0 0 0]  TranslationMethod=None  TranslationCartesianOffset=[0 0 0]  TranslationCartesianOffsetUnits=m  TranslationStandardAxis=+Z  TranslationStandardOffset=0  TranslationStandardOffsetUnits=m  TranslationROffset=0  TranslationROffsetUnits=m  TranslationThetaOffset=0  TranslationThetaOffsetUnits=deg  TranslationZOffset=0  TranslationZOffsetUnits=m
      settings: AttributesFormatString=|
      | %<RotationStandardAxis>
      | %<RotationAngle> deg
  Weld Joint2 : sm_lib/Joints/Weld Joint  Description=|  JointMode=Normal  CompositeWrenchDir=FollowerOnBase  CompositeWrenchFrame=BaseFrame  SenseConstraintForce=off  SenseConstraintTorque=off  SenseTotalForce=on  SenseTotalTorque=off
      | Total force
      | sensing
      settings: AttributesFormatString=%<Description>
  B : PMIOPort  Side=Left
  F : PMIOPort  Port=2  Side=Right
  Ni : Outport
  wires:
  Interpreted MATLAB Function/1 -> Dot Product/1
  Dot Product/1 -> Ni/1
  PS-Simulink Converter6/1 -> Interpreted MATLAB Function/1
  con/1 -> Dot Product/2
  connections:
  Weld Joint2/LConn1 -- Rigid Transform1/RConn1
  Flexible Cylindrical Beam1/LConn1 -- Weld Joint2/RConn1
  Rigid Transform1/LConn1 -- B/RConn1
  Rigid Transform2/RConn1 -- F/RConn1
  Flexible Cylindrical Beam1/RConn1 -- Rigid Transform2/LConn1
  Weld Joint2/RConn2 -- PS-Simulink Converter6/LConn1

== system Extended_Model_1_1/Subsystem6/Beam_3 ==
  note: Beam_C
  con : Inport
  Beam : sm_lib/Body Elements/Flexible Bodies/Beams/Flexible Cylindrical Beam  SectionType=Solid  Radius=d/2  RadiusUnits=m  Thickness=1  ThicknessUnits=mm  Length=l  LengthUnits=m  StiffnessAndInertiaType=CalculateFromGeometry  Density=Density  DensityUnits=kg/m^3  ModuliType=YoungsShear  YoungsModulus=E  YoungsModulusUnits=GPa  PoissonsRatio=0.28  ShearModulus=G  ShearModulusUnits=GPa  GeometricCentroid=[0 0]  GeometricCentroidUnits=m  BendingCentroid=[0 0]  BendingCentroidUnits=m  ShearCenter=[0 0]  ShearCenterUnits=m  AxialRigidity=1  AxialRigidityUnits=Pa*m^2  FlexuralRigidity=[1 1]  FlexuralRigidityUnits=Pa*m^4  CrossFlexuralRigidity=0  CrossFlexuralRigidityUnits=Pa*m^4  TorsionalRigidity=1  TorsionalRigidityUnits=Pa*m^4  CenterOfMass=[0 0]  CenterOfMassUnits=m  MassPerUnitLength=1  MassPerUnitLengthUnits=kg/m  MassMomentOfInertiaDensity=[1 1]  MassMomentOfInertiaDensityUnits=kg*m  MassProductOfInertiaDensity=0  MassProductOfInertiaDensityUnits=kg*m  DampingType=Proportional  ProportionalDampingAlpha=bm  ProportionalDampingAlphaUnits=1/s  ProportionalDampingBeta=bk  ProportionalDampingBetaUnits=s  UniformModalDampingRatio=0.01  NumElements=1  ReductionType=None  NumRetainedModes=1  GraphicType=FromGeometry  GraphicVisPropType=SimpleVisualProperties  GraphicDiffuseColor=[0.5 0.5 0.5]  GraphicOpacity=1.0  GraphicSpecularColor=[0.5 0.5 0.5 1.0]  GraphicAmbientColor=[0.15 0.15 0.15 1.0]  GraphicEmissiveColor=[0.0 0.0 0.0 1.0]  GraphicShininess=75  DoExposeZminFrame=on  DoExposeZmaxFrame=on  SerializedFrames=<Frames/>
      settings: AttributesFormatString=%<Description>
  Dot Product : DotProduct  OutDataTypeStr=Inherit: Inherit via internal rule
  Interpreted MATLAB Function : MATLABFcn  Description=u(3)  MATLABFcn=u(3)
      settings: AttributesFormatString=%<Description>
  PS-Simulink Converter6 : nesl_utility/PS-Simulink Converter  PhysicalDomain=network_engine_domain  SubClassName=ps_output  LeftPortType=input  RightPortType=output  PseudoPeriodic=off  Frequencies=[]  VectorFormat=inherit  Unit=1  AffineConversion=off
  Rigid Transform1 : sm_lib/Frames and Transforms/Rigid Transform  RotationMethod=StandardAxis  FollAlignAxisA=+X  BaseAlignAxisA=+Y  FollAlignAxisB=+Y  BaseAlignAxisB=+Z  RotationStandardAxis=+Y  RotationAngle=90  RotationAngleUnits=deg  RotationArbitraryAxis=[0 0 1]  RotationSequenceAxes=FollowerAxes  RotationSequence=XYX  RotationSequenceAngles=[0 0 0]  RotationSequenceAnglesUnits=deg  RotationMatrix=[1 0 0; 0 1 0; 0 0 1]  Quaternion=[1 0 0 0]  TranslationMethod=None  TranslationCartesianOffset=[0 0 0]  TranslationCartesianOffsetUnits=m  TranslationStandardAxis=+Z  TranslationStandardOffset=0  TranslationStandardOffsetUnits=m  TranslationROffset=0  TranslationROffsetUnits=m  TranslationThetaOffset=0  TranslationThetaOffsetUnits=deg  TranslationZOffset=0  TranslationZOffsetUnits=m
      settings: AttributesFormatString=|
      | %<RotationStandardAxis>
      | %<RotationAngle> deg
  Rigid Transform2 : sm_lib/Frames and Transforms/Rigid Transform  RotationMethod=StandardAxis  FollAlignAxisA=+X  BaseAlignAxisA=+Y  FollAlignAxisB=+Y  BaseAlignAxisB=+Z  RotationStandardAxis=+Y  RotationAngle=-90  RotationAngleUnits=deg  RotationArbitraryAxis=[0 0 1]  RotationSequenceAxes=FollowerAxes  RotationSequence=XYX  RotationSequenceAngles=[0 0 0]  RotationSequenceAnglesUnits=deg  RotationMatrix=[1 0 0; 0 1 0; 0 0 1]  Quaternion=[1 0 0 0]  TranslationMethod=None  TranslationCartesianOffset=[0 0 0]  TranslationCartesianOffsetUnits=m  TranslationStandardAxis=+Z  TranslationStandardOffset=0  TranslationStandardOffsetUnits=m  TranslationROffset=0  TranslationROffsetUnits=m  TranslationThetaOffset=0  TranslationThetaOffsetUnits=deg  TranslationZOffset=0  TranslationZOffsetUnits=m
      settings: AttributesFormatString=|
      | %<RotationStandardAxis>
      | %<RotationAngle> deg
  Weld Joint2 : sm_lib/Joints/Weld Joint  Description=|  JointMode=Normal  CompositeWrenchDir=FollowerOnBase  CompositeWrenchFrame=BaseFrame  SenseConstraintForce=off  SenseConstraintTorque=off  SenseTotalForce=on  SenseTotalTorque=off
      | Total force
      | sensing
      settings: AttributesFormatString=%<Description>
  B : PMIOPort  Side=Left
  F : PMIOPort  Port=2  Side=Right
  Ni : Outport
  wires:
  Interpreted MATLAB Function/1 -> Dot Product/1
  Dot Product/1 -> Ni/1
  con/1 -> Dot Product/2
  PS-Simulink Converter6/1 -> Interpreted MATLAB Function/1
  connections:
  Weld Joint2/RConn2 -- PS-Simulink Converter6/LConn1
  Rigid Transform1/LConn1 -- B/RConn1
  Beam/RConn1 -- Rigid Transform2/LConn1
  Rigid Transform2/RConn1 -- F/RConn1
  Weld Joint2/LConn1 -- Rigid Transform1/RConn1
  Beam/LConn1 -- Weld Joint2/RConn1
